simulink model "Flexible_Beam_SS_Static_Deflection"  (R2017a)
settings: Solver=ode23t  StartTime=0.0  StopTime=100  RelTol=1e-3  EnableMultiTasking=on
InitFcn:
  | if ~exist('linsys_beam_fixfree','var') ||~exist('linsys_beam_rotfree','var')
  |    load SS_Damping_1e7.mat
  |    disp('State Space Models does not exist in workspace, loading presaved SS models')
  | end
StopFcn:
  | disp(['Static Deflection is ' num2str(SS_Def.signals.values(end)) ' m'])
undefined symbols (not defined in the file): beam_wall, beam_width, density, element_length, gravity, num_elem
libraries: cstblocks x1
Description:
  | State Space Model of Cantilever Beam
  | 
  | Copyright 2014-2017 The MathWorks, Inc.
settings Model: Creator=psanghvi  LastModifiedBy=smiller
settings DataIOCC: LimitDataPoints=on  SaveFormat=Array
settings OptimizationCC: LifeSpan=inf
settings DebuggingCC: UnderspecifiedInitializationDetection=Classic  MergeDetectMultiDrivingBlocksExec=none  SolverPrmCheckMsg=warning  AllowSymbolicDim=off  SFUnexpectedBacktrackingDiag=warning  SFNoUnconditionalDefaultTransitionDiag=warning  SFExecutionAtInitializationDiag=none
settings HardwareCC: ProdBitPerPointer=32  ProdBitPerSizeT=32  ProdBitPerPtrDiffT=32  ProdLargestAtomicFloat=None  ProdIntDivRoundTo=Undefined  ProdEndianess=Unspecified  ProdWordSize=32  ProdHWDeviceType=32-bit Generic
settings ModelReferenceCC: PropagateSignalLabelsOutOfModel=off
settings GRTTargetCC: TargetLangStandard=C89/C90 (ANSI)  GeneratePreprocessorConditionals=Disable all
settings ConfigComp: CovMetricSettings=dw  CovHtmlReporting=on  CovSaveCumulativeToWorkspaceVar=on  CovSaveSingleToWorkspaceVar=on  CovExternalEMLEnable=off  CovSFcnEnable=off

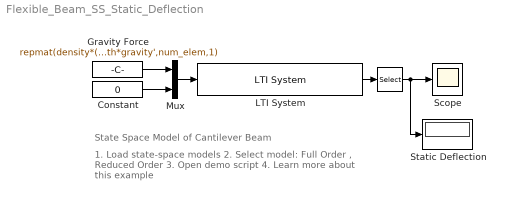
== system Flexible_Beam_SS_Static_Deflection ==
  note: State Space Model of Cantilever Beam
  note: 1. Load state-space models
      | 2. Select model: Full Order , Reduced Order
      | 3. Open demo script
      | 4. Learn more about this example
  "  " : Selector  InputPortWidth=num_elem+1  IndexOptions=Index vector (dialog)  Indices=num_elem+1  OutputSizes=1
  Constant : Constant  Value=0
  Gravity Force : Constant  Value=repmat(density*(beam_width^2- (beam_width-beam_wall*2)^2)*element_length*gravity',num_elem,1)
  LTI System : cstblocks/LTI System  sys=linsys_beam_fixfree  IC=[]
  Mux : Mux  Inputs=2
  Scope : Scope
  Static Deflection : Display
  wires:
  Constant/1 -> Mux/2
  Gravity Force/1 -> Mux/1
  Mux/1 -> LTI System/1
  LTI System/1 -> "  "/1
  "  "/1 -> Static Deflection/1, Scope/1
